simulink model "exp7"  (R2021a)
settings: Solver=VariableStepAuto  StartTime=0.0  StopTime=50  RelTol=1e-3
settings Model: Creator=jillianeuniceb.oliveros  LastModifiedBy=jillianeuniceb.oliveros

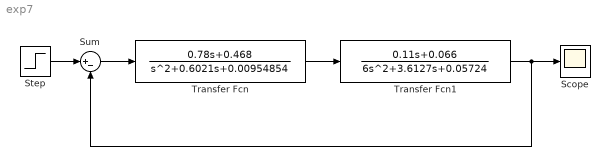
== system exp7 ==
  Scope : Scope
  Step : Step  Time=4  SampleTime=0
  Sum : Sum  Inputs=|+-
  Transfer Fcn : TransferFcn  Numerator=[0.78 0.468]  Denominator=[1 0.6021 0.00954854]
  Transfer Fcn1 : TransferFcn  Numerator=[0.11 0.066]  Denominator=[6 3.6127 0.05724]
  wires:
  Transfer Fcn/1 -> Transfer Fcn1/1
  Sum/1 -> Transfer Fcn/1
  Step/1 -> Sum/1
  Transfer Fcn1/1 -> Sum/2, Scope/1
